simulink model "Nicholas_Noise_SineWave"  (R2021b)
settings: Solver=VariableStepAuto  StartTime=0.0  StopTime=5  RelTol=1e-3
settings Model: Creator=NicholasYe  LastModifiedBy=NicholasYe

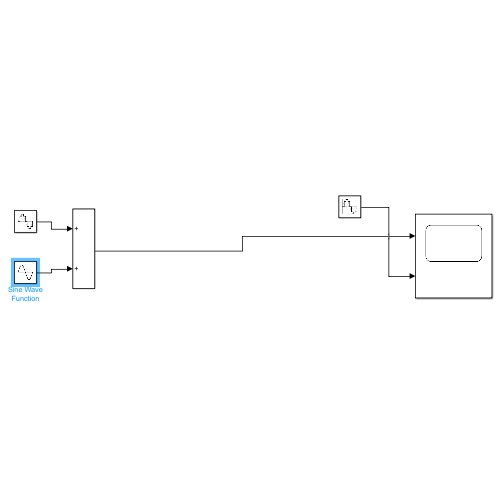
[thumbnail: Simulink's stored preview of the top-level diagram]
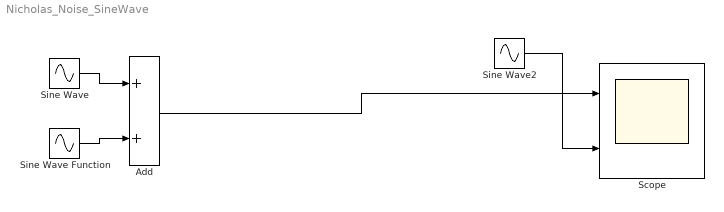
== system Nicholas_Noise_SineWave ==
  Add : Sum
  Scope : Scope  NumInputPorts=2
  Sine Wave : Sin  Amplitude=220  Frequency=100*pi  SampleTime=1e-6
  Sine Wave Function : Sin  Amplitude=30  Frequency=100*pi  SampleTime=0
  Sine Wave2 : Sin  Amplitude=220  Frequency=100*pi  SampleTime=1e-6
  wires:
  Sine Wave/1 -> Add/1
  Add/1 -> Scope/1
  Sine Wave2/1 -> Scope/2
  Sine Wave Function/1 -> Add/2
